simulink model "fxpdemo_sfun_user_prodsum"  (Simulink 5.0)
settings: Solver=FixedStepDiscrete  StartTime=0.0  StopTime=0.2  FixedStep=0.001  RelTol=1e-3
libraries: fixpt_lib_4 x3, simulink x2
settings Model: Creator=andyb  LastModifiedBy=andyb  ExtModeAutoUpdateStatusClock=off  ParameterPrecisionLossMsg=none  RTWInlineParameters=on  RTWOptions="-aEnforceIntegerDowncast=1 -aExtMode=0 -aExtModeTesting=0 -aFoldNonRolledExpr=1 -aForceParamTrailComments=0 -aGenerateComments=1 -aGenerateFullHeader=1 -aGenerateReport=1 -aIgnoreCustomStorageClasses=1 -aIncDataTypeInIds=0 -aIncHierarchyInIds=0 -aInlineInvariantSignals=0 -aInlineParameters=1 -aInlinedPrmAccess=\"Literals\" -aLocalBlockOutputs=1 -aLogVarNameModifier=\"rt_\" -aMaxRTWIdLen=31 -aPrefixModelToSubsysFcnNames=1 -aRTWVerbose=1 -aRollThreshold=5 -aShowEliminatedStatements=0"

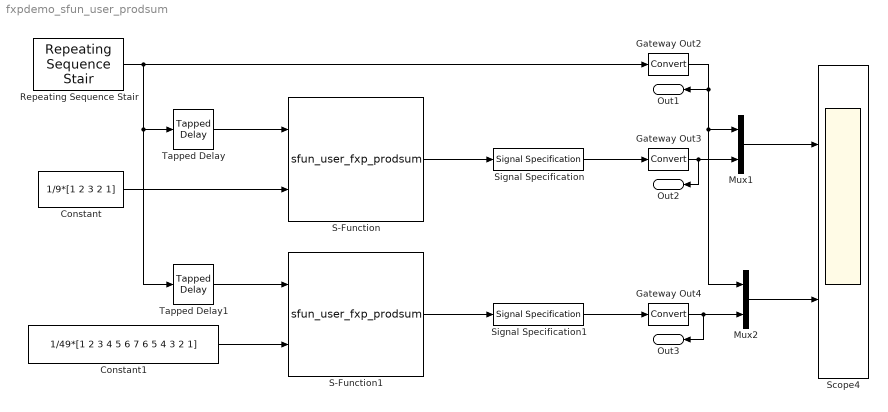
== system fxpdemo_sfun_user_prodsum ==
  Constant : Constant  Value=1/9*[1 2 3 2 1]  ShowAdditionalParam=on  OutDataTypeMode=Specify via dialog  ConRadixGroup=Best Precision: Vector-wise  OutScaling=2^-10
  Constant1 : Constant  Value=1/49*[1 2 3 4 5 6 7 6 5 4 3 2 1]  ShowAdditionalParam=on  OutDataTypeMode=Specify via dialog  OutScaling=2^-16
  Gateway Out2 : DataTypeConversion  DataType=double
  Gateway Out3 : DataTypeConversion  DataType=double
  Gateway Out4 : DataTypeConversion  DataType=double
  Mux1 : Mux  Inputs=2
  Mux2 : Mux  Inputs=2
  Repeating Sequence Stair : fixpt_lib_4/Sources/Repeating Sequence Stair  OutValues=5*sin(10*2*pi*(0:200)/200)  tsamp=-1  OutputDataTypeScalingMode=Specify via dialog  OutDataType=sfix(16)  OutScaling=2^-12  ConRadixGroup=Best Precision: Vector-wise
  S-Function : S-Function  FunctionName=sfun_user_fxp_prodsum
  S-Function1 : S-Function  FunctionName=sfun_user_fxp_prodsum
  Scope4 : Scope  NumInputPorts=2
      settings: TimeRange=0.2  YMin=-5~-5  YMax=5~5  SaveName=ScopeData3
  Signal Specification : simulink/Signal Attributes/Signal Specification  D=-1  Ts=-1  DataType=Specify via dialog  OutDataType=sfix(16)  OutScaling=2^-12
      settings: SignalType=auto  SamplingMode=auto
  Signal Specification1 : simulink/Signal Attributes/Signal Specification  D=-1  Ts=-1  DataType=Specify via dialog  OutDataType=sfix(16)  OutScaling=2^-10
      settings: SignalType=auto  SamplingMode=auto
  Tapped Delay : fixpt_lib_4/Delays & Holds/Tapped Delay  vinit=0.0  samptime=-1  NumDelays=5  DelayOrder=Oldest
  Tapped Delay1 : fixpt_lib_4/Delays & Holds/Tapped Delay  vinit=0.0  samptime=-1  NumDelays=13  DelayOrder=Oldest
  Out1 : Outport  Orientation=left
  Out2 : Outport  Orientation=left  Port=2
  Out3 : Outport  Orientation=left  Port=3
  wires:
  Mux1/1 -> Scope4/1
  Gateway Out3/1 -> Mux1/2, Out2/1
  S-Function/1 -> Signal Specification/1
  Constant/1 -> S-Function/2
  Tapped Delay/1 -> S-Function/1
  Signal Specification/1 -> Gateway Out3/1
  Mux2/1 -> Scope4/2
  Gateway Out4/1 -> Mux2/2, Out3/1
  S-Function1/1 -> Signal Specification1/1
  Signal Specification1/1 -> Gateway Out4/1
  Repeating Sequence Stair/1 -> Gateway Out2/1, Tapped Delay/1, Tapped Delay1/1
  Tapped Delay1/1 -> S-Function1/1
  Constant1/1 -> S-Function1/2
  Gateway Out2/1 -> Out1/1, Mux1/1, Mux2/1
